simulink model "model"  (R2020b)
settings: Solver=VariableStepAuto  StartTime=0.0  StopTime=15.0  RelTol=1e-3
values from neighbouring files (symbols this model uses):
  a = 2    [cw1.m]    (also in model_s.m)
  b = 1    [cw1.m]    (also in model_s.m)
settings Model: Creator=stasz  LastModifiedBy=stasz

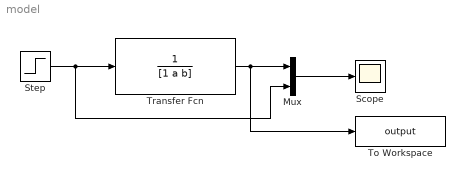
== system model ==
  Mux : Mux  Inputs=2
  Scope : Scope
  Step : Step  SampleTime=0
  To Workspace : ToWorkspace  VariableName=output  SaveFormat=Timeseries  SampleTime=-1
  Transfer Fcn : TransferFcn  Denominator=[1 a b]
  wires:
  Transfer Fcn/1 -> Mux/1, To Workspace/1
  Mux/1 -> Scope/1
  Step/1 -> Mux/2, Transfer Fcn/1
